simulink model "model_const_angle"  (R2022a)
settings: Solver=VariableStepAuto  StartTime=0.0  StopTime=1000  RelTol=1e-3
values from neighbouring files (symbols this model uses):
  angle_init = abs(pi/2*(v_init-128)/128)    [in.m]
  drain_area = pi*(drain_d^2)/4    (= 7.85398163397e-05)    [in.m]
  g = 9.8    [in.m]
  input_5litre = 11/12    (= 0.916666666667)    [in.m]
  pump_max_speed = 1/10000    (= 0.0001)    [in.m]
  pump_switch = 0.5    [in.m]
  pwm_bits = 8    [in.m]
  pwm_T = 2^pwm_bits/mc_freq    (= 1.6e-05)    [in.m]
  target_area = target_V/target_h    (= 0.025)    [in.m]
  theta0 = asin(1 - pump_speed/drain_area/sqrt(2*g*target_h))    [in.m]
  v_init = 0    [in.m]
libraries: simulink x1
settings Model: Creator=ilyas  LastModifiedBy=ilyas

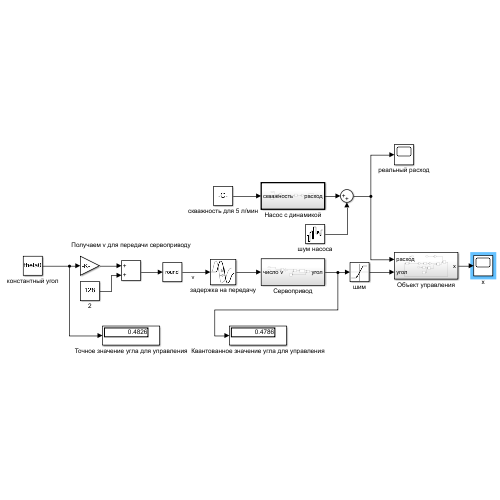
[thumbnail: Simulink's stored preview of the top-level diagram]
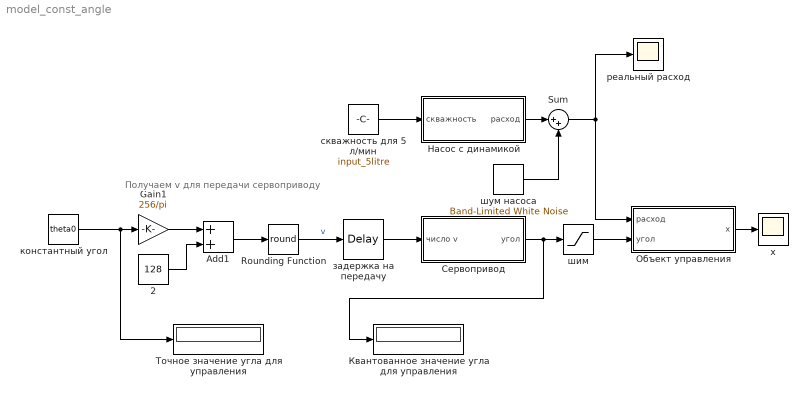
== system model_const_angle ==
  note: Получаем v для передачи сервоприводу
  2 : Constant  Value=128
  Add1 : Sum
  Gain1 : Gain  Gain=256/pi
  Rounding Function : Rounding  Operator=round
  Sum : Sum  Inputs=|++
  Квантованное значение угла для управления : Display
  Насос с динамикой : Subsystem  TreatAsAtomicUnit=on
  Объект управления : Subsystem
  Сервопривод : Subsystem
  Точное значение угла для управления : Display
  задержка на передачу : TransportDelay  DelayTime=56/9600  InitialOutput=v_init
  константный угол : Constant  Value=theta0
  реальный расход : Scope
  скважность для 5 л/мин : Constant  Value=input_5litre
  х : Scope
  шим : Saturate  UpperLimit=pi  LowerLimit=-pi
  шум насоса : simulink/Sources/Band-Limited White Noise  Cov=[0.0000000000001]  Ts=0.1  seed=[23341]
  wires:
  скважность для 5 л/мин/1 -> Насос с динамикой/1(скважность)
  Насос с динамикой/1(расход) -> Sum/1
  шум насоса/1 -> Sum/2
  задержка на передачу/1 -> Сервопривод/1(число v)
  Rounding Function/1 -> задержка на передачу/1  "v"
  Gain1/1 -> Add1/1
  2/1 -> Add1/2
  Add1/1 -> Rounding Function/1
  Сервопривод/1(угол) -> шим/1, Квантованное значение угла для управления/1
  константный угол/1 -> Точное значение угла для управления/1, Gain1/1
  Sum/1 -> реальный расход/1, Объект управления/1(расход)
  Объект управления/1(х) -> х/1
  шим/1 -> Объект управления/2(угол)

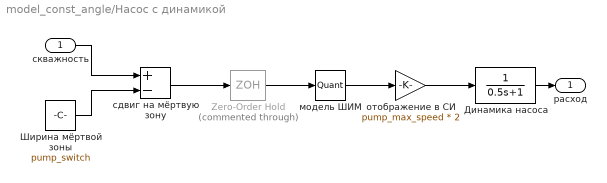
== system model_const_angle/Насос с динамикой ==
  скважность : Inport
  Zero-Order Hold : ZeroOrderHold  Commented=through  SampleTime=pwm_T
  Динамика насоса : TransferFcn  Denominator=[0.5 1]
  Ширина мёртвой зоны : Constant  Value=pump_switch
  модель ШИМ : Quantizer  QuantizationInterval=0.25/2^pwm_bits
  отображение в СИ : Gain  Gain=pump_max_speed * 2
  сдвиг на мёртвую зону : Sum  Inputs=+-
  расход : Outport
  wires:
  сдвиг на мёртвую зону/1 -> Zero-Order Hold/1
  скважность/1 -> сдвиг на мёртвую зону/1
  Ширина мёртвой зоны/1 -> сдвиг на мёртвую зону/2
  модель ШИМ/1 -> отображение в СИ/1
  отображение в СИ/1 -> Динамика насоса/1
  Динамика насоса/1 -> расход/1
  Zero-Order Hold/1 -> модель ШИМ/1

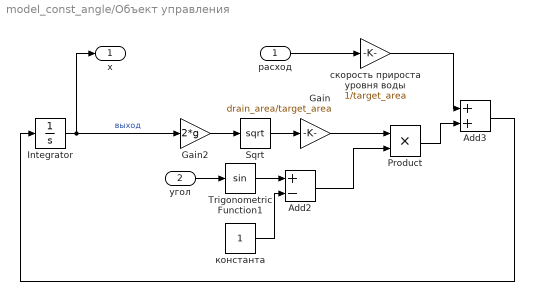
== system model_const_angle/Объект управления ==
  расход : Inport
  угол : Inport  Port=2
  Add2 : Sum  Inputs=+-
  Add3 : Sum
  Gain : Gain  Gain=drain_area/target_area
  Gain2 : Gain  Gain=2*g
  Integrator : Integrator
  Product : Product
  Sqrt : Sqrt
  Trigonometric Function1 : Trigonometry
  константа : Constant
  скорость прироста уровня воды : Gain  Gain=1/target_area
  х : Outport
  wires:
  скорость прироста уровня воды/1 -> Add3/1
  Gain2/1 -> Sqrt/1
  Add3/1 -> Integrator/1
  Add2/1 -> Product/2
  Product/1 -> Add3/2
  константа/1 -> Add2/2
  расход/1 -> скорость прироста уровня воды/1
  Integrator/1 -> Gain2/1, х/1  "выход"
  угол/1 -> Trigonometric Function1/1
  Trigonometric Function1/1 -> Add2/1
  Sqrt/1 -> Gain/1
  Gain/1 -> Product/1

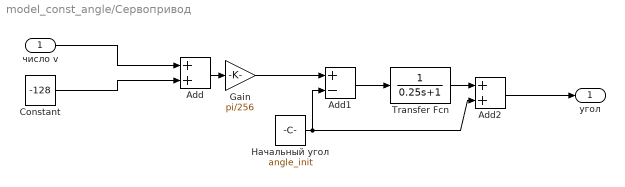
== system model_const_angle/Сервопривод ==
  число v : Inport
  Add : Sum
  Add1 : Sum  Inputs=+-
  Add2 : Sum
  Constant : Constant  Value=-128
  Gain : Gain  Gain=pi/256
  Transfer Fcn : TransferFcn  Denominator=[0.25 1]
  Начальный угол : Constant  Value=angle_init
  угол : Outport
  wires:
  Constant/1 -> Add/2
  Add/1 -> Gain/1
  число v/1 -> Add/1
  Transfer Fcn/1 -> Add2/1
  Начальный угол/1 -> Add1/2, Add2/2
  Add1/1 -> Transfer Fcn/1
  Gain/1 -> Add1/1
  Add2/1 -> угол/1
